simulink model "testfcall_child_3"  (Simulink 9.2)
settings: Solver=FixedStepDiscrete  StartTime=0.0  StopTime=10.0  FixedStep=1  RelTol=1e-3  EnableMultiTasking=on
settings Model: Creator=smorikaw  LastModifiedBy=E00026
settings OptimizationCC: DefaultParameterBehavior=Inlined  ExpressionDepthLimit=2147483647
settings DebuggingCC: UnderspecifiedInitializationDetection=Simplified  MergeDetectMultiDrivingBlocksExec=error  SolverPrmCheckMsg=warning
settings ModelReferenceCC: UpdateModelReferenceTargets=IfOutOfDate  ModelReferenceNumInstancesAllowed=Single

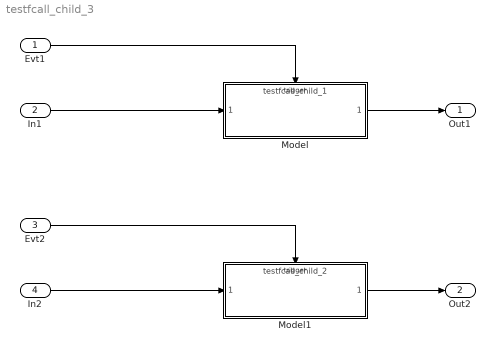
== system testfcall_child_3 ==
  Evt1 : Inport  Priority=2  OutputFunctionCall=on
  In1 : Inport  Port=2
  Evt2 : Inport  Priority=1  Port=3  OutputFunctionCall=on
  In2 : Inport  Port=4
  Model : ModelReference  ModelNameDialog=testfcall_child_1  SimulationMode=Normal  ModelReferenceVersion=1.28  TriggerPortName=function  TriggerPortTriggerType=function-call  TriggerPortStatesWhenEnabling=held
  Model1 : ModelReference  ModelNameDialog=testfcall_child_2.mdl  SimulationMode=Normal  ModelReferenceVersion=1.30  TriggerPortName=function  TriggerPortTriggerType=function-call  TriggerPortStatesWhenEnabling=held
  Out1 : Outport
  Out2 : Outport  Port=2
  wires:
  In1/1 -> Model/1
  Model/1 -> Out1/1
  In2/1 -> Model1/1
  Model1/1 -> Out2/1
  Evt1/1 -> Model/Trigger
  Evt2/1 -> Model1/Trigger
